simulink model "sfcndemo_sfun_atol"  (Simulink 6.0)
settings: Solver=ode45  StartTime=0.0  StopTime=20.0  RelTol=1e-3  AbsTol=1.0e-9
settings Model: Creator=The MathWorks Inc.  LastModifiedBy=batserve  ExtModeAutoUpdateStatusClock=off
settings DataIOCC: SaveFormat=StructureWithTime  SaveState=on
settings OptimizationCC: BlockReduction=off  BooleanDataType=off
settings DebuggingCC: CheckExecutionContextPreStartOutputMsg=on  CheckExecutionContextRuntimeOutputMsg=on  SolverPrmCheckMsg=none
settings HardwareCC: TargetUnknown=on

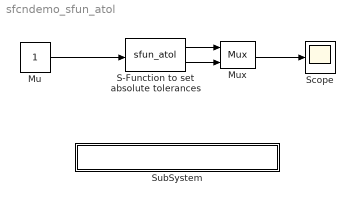
== system sfcndemo_sfun_atol ==
  Mu : Constant
  Mux : Mux  Inputs=2
  S-Function to set absolute tolerances : S-Function  FunctionName=sfun_atol  Parameters=abstol0 abstol1  mask{abstol0=1.0e-6, abstol1=1.0e-6}
      mask prompts: abstol0 "AbsTol[0]:"; abstol1 "AbsTol[1]"
      mask help: This S-function allows the user to set the absolute tolerance for each continuous state. In this case there are two continous states whose absolute tolerances can be set using parameters.
      mask Display: disp('sfun_atol')
  Scope : Scope
  SubSystem : Subsystem  PropExecContextAcrossSSBoundary=on
      settings: OpenFcn=edit(fullfile(matlabroot,'simulink','src','sfun_atol.c'))
      mask Display: disp('matlabroot\simulink\src\sfun_atol.c');
  wires:
  Mu/1 -> S-Function to set absolute tolerances/1
  S-Function to set absolute tolerances/1 -> Mux/1
  S-Function to set absolute tolerances/2 -> Mux/2
  Mux/1 -> Scope/1

== system sfcndemo_sfun_atol/SubSystem ==
